simulink model "L4A2_e_simu"  (R2021b)
settings: Solver=VariableStepAuto  StartTime=0.0  StopTime=60  MaxStep=0.0001  RelTol=1e-3
values from neighbouring files (symbols this model uses):
  K_r = Verstaerkungsfaktoren(i)    [L4A2.m]    (also in L4A2_c2.m; L4A2_d.m; L4A2_e.m)
settings Model: Creator=tobia  LastModifiedBy=tobia

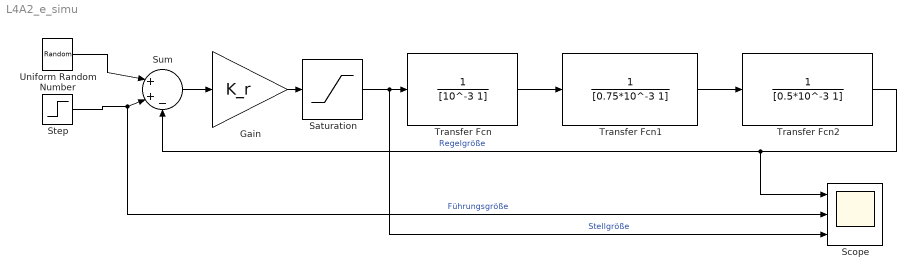
== system L4A2_e_simu ==
  Gain : Gain  Gain=K_r
  Saturation : Saturate  UpperLimit=12  LowerLimit=-12
  Scope : Scope  NumInputPorts=3
  Step : Step  Time=0  After=0  SampleTime=0
  Sum : Sum  Inputs=|++-
  Transfer Fcn : TransferFcn  Denominator=[10^-3 1]
  Transfer Fcn1 : TransferFcn  Denominator=[0.75*10^-3 1]
  Transfer Fcn2 : TransferFcn  Denominator=[0.5*10^-3 1]
  Uniform Random Number : UniformRandomNumber  Minimum=-0.01  Maximum=0.01  SampleTime=0.001
  wires:
  Transfer Fcn/1 -> Transfer Fcn1/1
  Transfer Fcn1/1 -> Transfer Fcn2/1
  Gain/1 -> Saturation/1
  Saturation/1 -> Scope/3, Transfer Fcn/1  "Stellgröße"
  Transfer Fcn2/1 -> Sum/3, Scope/1  "Regelgröße"
  Sum/1 -> Gain/1
  Step/1 -> Sum/2, Scope/2  "Führungsgröße"
  Uniform Random Number/1 -> Sum/1
